simulink model "uz_pmsm_model_6ph_dqxy"  (R2024b)
settings: Solver=FixedStepAuto  StartTime=0.0  StopTime=0.5  RelTol=1e-3
PreLoadFcn:
  | uz_pmsm_model_6ph_dqxy_init_parameter
values from neighbouring files (symbols this model uses):
  friction_coefficient = 0.001    [uz_pmsm_model_6ph_dqxy_init_parameter.m]
  inertia = 0.001    [uz_pmsm_model_6ph_dqxy_init_parameter.m]
  k_i_d = R_1/(2*tau_sum)    (= 10500)    [uz_pmsm_model_6ph_dqxy_init_parameter.m]
  k_i_x = R_1/(2*tau_sum)    (= 10500)    [uz_pmsm_model_6ph_dqxy_init_parameter.m]
  k_i_y = R_1/(2*tau_sum)    (= 10500)    [uz_pmsm_model_6ph_dqxy_init_parameter.m]
  k_p_d = L_d/(2*tau_sum)    (= 150)    [uz_pmsm_model_6ph_dqxy_init_parameter.m]
  k_p_q = L_q/(2*tau_sum)    (= 250)    [uz_pmsm_model_6ph_dqxy_init_parameter.m]
  k_p_x = L_x/(2*tau_sum)    (= 15)    [uz_pmsm_model_6ph_dqxy_init_parameter.m]
  k_p_y = L_y/(2*tau_sum)    (= 25)    [uz_pmsm_model_6ph_dqxy_init_parameter.m]
  L_d = 30e-3    (= 0.03)    [uz_pmsm_model_6ph_dqxy_init_parameter.m]
  L_q = 50e-3    (= 0.05)    [uz_pmsm_model_6ph_dqxy_init_parameter.m]
  L_x = 30e-4    (= 0.003)    [uz_pmsm_model_6ph_dqxy_init_parameter.m]
  L_y = 50e-4    (= 0.005)    [uz_pmsm_model_6ph_dqxy_init_parameter.m]
  polepair = 2    [uz_pmsm_model_6ph_dqxy_init_parameter.m]
  psi_pm = 0.05    [uz_pmsm_model_6ph_dqxy_init_parameter.m]
  R_1 = 2.1    [uz_pmsm_model_6ph_dqxy_init_parameter.m]
  setpoint_step = 10.0    (= 10)    [uz_pmsm_model_6ph_dqxy_init_parameter.m]
  simulate_mechanical = true    [uz_pmsm_model_6ph_dqxy_init_parameter.m]
  simulate_open_loop = true    [uz_pmsm_model_6ph_dqxy_init_parameter.m]
  static_friction_torque = 0.01    [uz_pmsm_model_6ph_dqxy_init_parameter.m]
  ts = 1/2e6    (= 5e-07)    [uz_pmsm_model_6ph_dqxy_init_parameter.m]
libraries: slpidlib x4
settings Model: DataTypeOverride=Off  Creator=ts  LastModifiedBy=hufnagelde
settings SolverCC: AlgebraicLoopSolver=TrustRegion  AutoInsertRateTranBlk=on
settings DataIOCC: LimitDataPoints=on  SaveOutput=off  SaveTime=off
settings OptimizationCC: BlockReduction=off  ConditionallyExecuteInputs=off  DefaultParameterBehavior=Inlined  LifeSpan=inf
settings DebuggingCC: AlgebraicLoopMsg=error  SingleTaskRateTransMsg=error  UnconnectedInputMsg=warning  UnconnectedOutputMsg=warning  UnconnectedLineMsg=warning  AllowSymbolicDim=off  StrictBusMsg=ErrorOnBusTreatedAsVector  SFUnexpectedBacktrackingDiag=warning  SFNoUnconditionalDefaultTransitionDiag=warning  SFExecutionAtInitializationDiag=none  ArithmeticOperatorsInVariantConditions=warning
settings HardwareCC: ProdBitPerPointer=32  ProdBitPerSizeT=32  ProdBitPerPtrDiffT=32  ProdLargestAtomicFloat=None  ProdIntDivRoundTo=Undefined  ProdEndianess=Unspecified  ProdWordSize=32  ProdHWDeviceType=ASIC/FPGA->ASIC/FPGA  ProdEqTarget=off
settings ModelReferenceCC: EnableRefExpFcnMdlSchedulingChecks=on
settings SFSimCC: SimUseLocalCustomCode=off  CustomCodeUndefinedFunction=UseInterfaceOnly
settings RTWCC: RTWUseLocalCustomCode=off  GPUComputeCapability=3.5  DLArmComputeVersion=19.05
settings CodeAppCC: StateflowObjectComments=on
settings GRTTargetCC: TargetLangStandard=C89/C90 (ANSI)
settings ConfigComp: CovScope=ReferencedModels  CovMetricSettings=dw  CovSaveCumulativeToWorkspaceVar=on  CovSaveSingleToWorkspaceVar=on  CovExternalEMLEnable=off  CovSFcnEnable=off

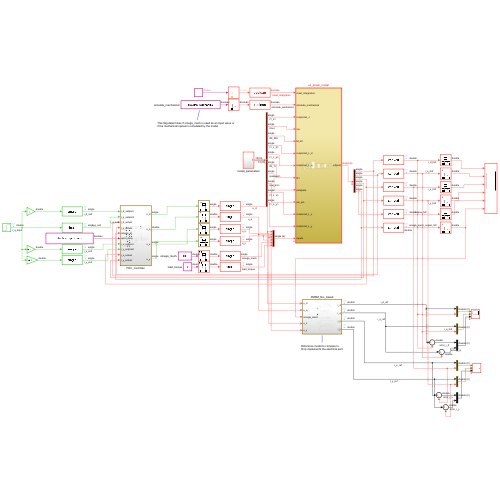
[thumbnail: Simulink's stored preview of the top-level diagram]
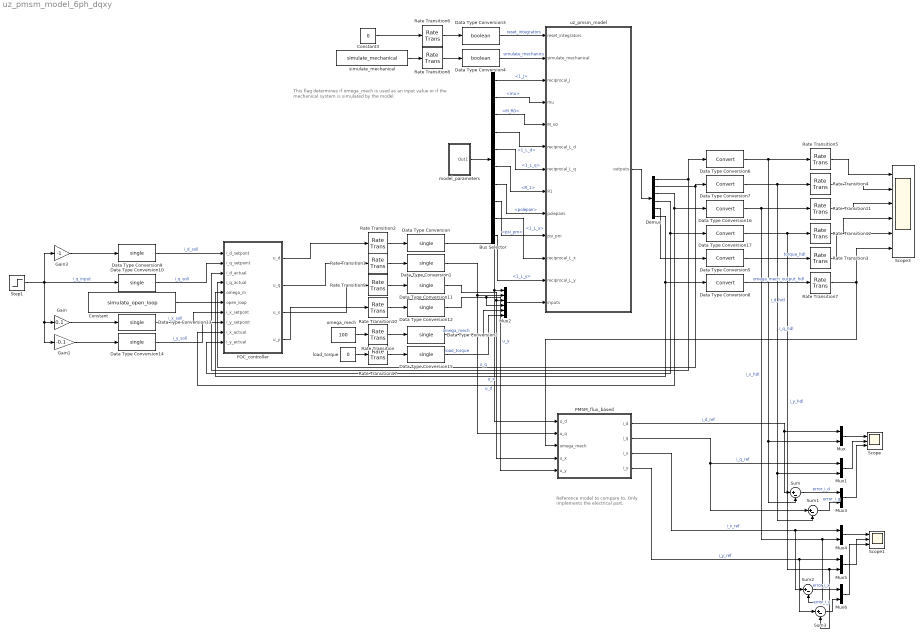
== system uz_pmsm_model_6ph_dqxy ==
  note: Reference model to compare to.
      | Only implements the electrical part.
  note: This flag determines if omega_mech is used as an input value or
      | if the mechanical system is simulated by the model
  Bus Selector : BusSelector  OutputSignals=1_J,mu,M_R0,1_L_d,1_L_q,R_1,polepair,psi_pm,1_L_x,1_L_y
  Constant : Constant  Value=simulate_open_loop
  Constant3 : Constant  Value=0
  Data Type Conversion{,1..2,9..15} (10 alike) : DataTypeConversion  OutDataTypeStr=single  SaturateOnIntegerOverflow=off  RndMeth=Floor
  Data Type Conversion{5..8,16..17} (6 alike) : DataTypeConversion  SaturateOnIntegerOverflow=off  RndMeth=Floor
  Data Type Conversion3 : DataTypeConversion  OutDataTypeStr=boolean  SaturateOnIntegerOverflow=off  RndMeth=Floor
  Data Type Conversion4 : DataTypeConversion  OutDataTypeStr=boolean  SaturateOnIntegerOverflow=off  RndMeth=Floor
  Demux : Demux  Outputs=6
  FOC_controller : Subsystem
  Gain : Gain  Gain=0.1
  Gain1 : Gain  Gain=-0.1
  Gain3 : Gain  Gain=-1
  Mux{,1,3..6} (6 alike) : Mux  Inputs=2
  Mux2 : Mux  Inputs=6
  PMSM_flux_based : Subsystem
  Rate Transition{,1..2,6,8..10,17} (8 alike) : RateTransition  OutPortSampleTime=ts
  Rate Transition{3..5,7,11..12} (6 alike) : RateTransition
  Scope : Scope  NumInputPorts=3
  Scope1 : Scope  NumInputPorts=3
  Scope3 : Scope  NumInputPorts=6
  Step1 : Step  Time=0.2  After=setpoint_step
  Sum{,1..3} (4 alike) : Sum  Inputs=|+-
  load_torque : Constant  Value=0
  model_parameters : Subsystem
  omega_mech : Constant  Value=100
  simulate_mechanical : Constant  Value=simulate_mechanical
  uz_pmsm_model : Subsystem  TreatAsAtomicUnit=on
  wires:
  Rate Transition/1 -> Data Type Conversion2/1
  Data Type Conversion6/1 -> Mux/2, Sum/2, Rate Transition5/1  "i_d_hdl"
  Data Type Conversion7/1 -> Mux1/2, Sum1/2, Rate Transition4/1  "i_q_hdl"
  Data Type Conversion5/1 -> Rate Transition3/1  "torque_hdl"
  Rate Transition4/1 -> Scope3/2
  Rate Transition5/1 -> Scope3/1
  Rate Transition3/1 -> Scope3/5
  Rate Transition6/1 -> Data Type Conversion3/1
  Constant3/1 -> Rate Transition6/1
  Rate Transition8/1 -> Data Type Conversion4/1
  simulate_mechanical/1 -> Rate Transition8/1
  Data Type Conversion3/1 -> uz_pmsm_model/1(reset_integrators)  "reset_integrators"
  Data Type Conversion4/1 -> uz_pmsm_model/2(simulate_mechanical)  "simulate_mechanics"
  load_torque/1 -> Rate Transition17/1
  Rate Transition17/1 -> Data Type Conversion15/1
  Mux/1 -> Scope/1
  Mux1/1 -> Scope/2
  PMSM_flux_based/2(i_q) -> Mux1/1, Sum1/1  "i_q_ref"
  PMSM_flux_based/1(i_d) -> Mux/1, Sum/1  "i_d_ref"
  Data Type Conversion8/1 -> Rate Transition7/1  "omega_mech_output_hdl"
  Rate Transition7/1 -> PMSM_flux_based/3(omega_mech), Scope3/6
  Bus Selector/1 -> uz_pmsm_model/3(reciprocal_J)  "<1_J>"
  Bus Selector/2 -> uz_pmsm_model/4(mu)  "<mu>"
  Bus Selector/3 -> uz_pmsm_model/5(M_n0)  "<M_R0>"
  Bus Selector/4 -> uz_pmsm_model/6(reciprocal_L_d)  "<1_L_d>"
  Bus Selector/5 -> uz_pmsm_model/7(reciprocal_L_q)  "<1_L_q>"
  Bus Selector/6 -> uz_pmsm_model/8(R1)  "<R_1>"
  Bus Selector/7 -> uz_pmsm_model/9(polepairs)  "<polepair>"
  Bus Selector/8 -> uz_pmsm_model/10(psi_pm)  "<psi_pm>"
  model_parameters/1(Out1) -> Bus Selector/1
  Sum/1 -> Mux3/1  "error_i_d"
  Sum1/1 -> Mux3/2  "error_i_q"
  Mux3/1 -> Scope/3
  Step1/1 -> Gain1/1, Gain/1, Gain3/1, Data Type Conversion10/1  "i_q_input"
  Demux/5 -> Data Type Conversion5/1
  Gain3/1 -> Data Type Conversion9/1
  Demux/1 -> FOC_controller/3(i_d_actual), Data Type Conversion6/1
  Demux/6 -> FOC_controller/5(omega_m), Data Type Conversion8/1
  Demux/2 -> FOC_controller/4(i_q_actual), Data Type Conversion7/1
  Data Type Conversion/1 -> PMSM_flux_based/1(u_d), Mux2/1  "u_d"
  Data Type Conversion1/1 -> PMSM_flux_based/2(u_q), Mux2/2  "u_q"
  Data Type Conversion15/1 -> Mux2/6  "load_torque"
  Data Type Conversion2/1 -> Mux2/5  "omega_mech"
  Mux2/1 -> uz_pmsm_model/13(inputs)
  uz_pmsm_model/1(outputs) -> Demux/1
  Data Type Conversion9/1 -> FOC_controller/1(i_d_setpont)  "i_d_soll"
  Data Type Conversion10/1 -> FOC_controller/2(i_q_setpoint)  "i_q_soll"
  omega_mech/1 -> Rate Transition/1
  Constant/1 -> FOC_controller/6(open_loop)
  Rate Transition9/1 -> Data Type Conversion11/1
  Rate Transition10/1 -> Data Type Conversion12/1
  Rate Transition1/1 -> Data Type Conversion1/1
  Rate Transition2/1 -> Data Type Conversion/1
  FOC_controller/1(u_d) -> Rate Transition2/1
  FOC_controller/2(u_q) -> Rate Transition1/1
  FOC_controller/3(u_x) -> Rate Transition9/1
  FOC_controller/4(u_y) -> Rate Transition10/1
  Data Type Conversion11/1 -> PMSM_flux_based/4(u_x), Mux2/3  "u_x"
  Data Type Conversion12/1 -> PMSM_flux_based/5(u_y), Mux2/4  "u_y"
  Gain1/1 -> Data Type Conversion14/1
  Gain/1 -> Data Type Conversion13/1
  Data Type Conversion13/1 -> FOC_controller/7(i_x_setpont)  "i_x_soll"
  Data Type Conversion14/1 -> FOC_controller/8(i_y_setpoint)  "i_y_soll"
  Data Type Conversion16/1 -> Sum2/2, Mux4/2, Rate Transition11/1  "i_x_hdl"
  Rate Transition11/1 -> Scope3/3
  Demux/3 -> FOC_controller/9(i_x_actual), Data Type Conversion16/1
  Data Type Conversion17/1 -> Sum3/2, Mux5/2, Rate Transition12/1  "i_y_hdl"
  Rate Transition12/1 -> Scope3/4
  Demux/4 -> FOC_controller/10(i_y_actual), Data Type Conversion17/1
  Mux4/1 -> Scope1/1
  PMSM_flux_based/3(i_x) -> Sum2/1, Mux4/1  "i_x_ref"
  PMSM_flux_based/4(i_y) -> Mux5/1, Sum3/1  "i_y_ref"
  Mux5/1 -> Scope1/2
  Sum2/1 -> Mux6/1  "error_i_x"
  Sum3/1 -> Mux6/2  "error_i_y"
  Mux6/1 -> Scope1/3
  Bus Selector/9 -> uz_pmsm_model/11(reciprocal_L_x)  "<1_L_x>"
  Bus Selector/10 -> uz_pmsm_model/12(reciprocal_L_y)  "<1_L_y>"

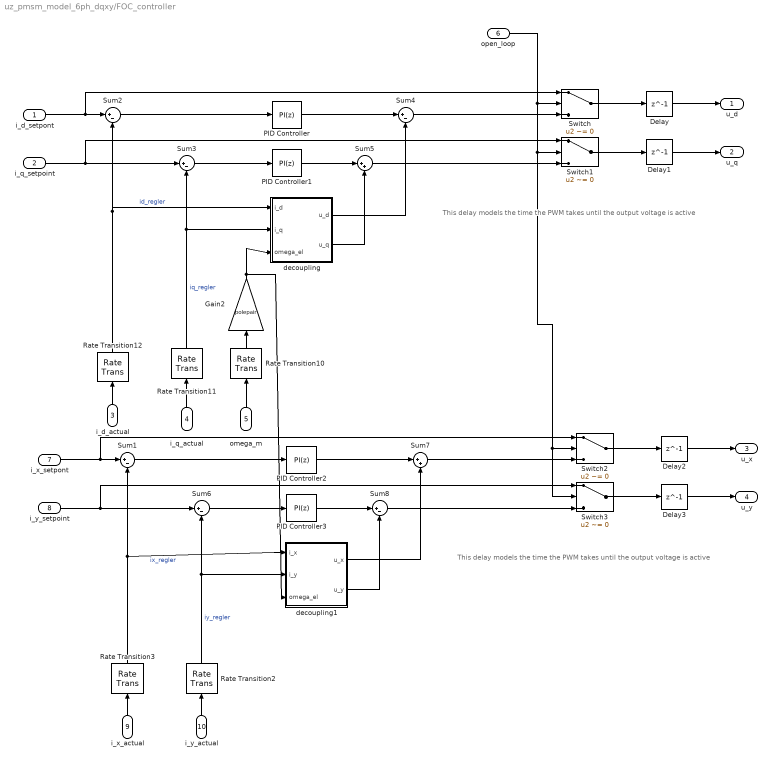
== system uz_pmsm_model_6ph_dqxy/FOC_controller ==
  note: This delay models the time the PWM takes until the output voltage is active
  note: This delay models the time the PWM takes until the output voltage is active
  i_d_setpont : Inport
  i_q_setpoint : Inport  Port=2
  i_d_actual : Inport  Port=3
  i_q_actual : Inport  Port=4
  omega_m : Inport  Port=5
  open_loop : Inport  Port=6
  i_x_setpont : Inport  Port=7
  i_y_setpoint : Inport  Port=8
  i_x_actual : Inport  Port=9
  i_y_actual : Inport  Port=10
  Delay{,1..3} (4 alike) : Delay  DelayLength=1
  Gain2 : Gain  Gain=polepair
  PID Controller : slpidlib/PID Controller  Controller=PI  Form=Parallel  TimeDomain=Discrete-time  UseExternalTs=off  SampleTime=-1  IntegratorMethod=Forward Euler  FilterMethod=Forward Euler  ControllerParametersSource=internal  P=k_p_d  I=k_i_d  UseKiTs=off  D=0  UseExternalDerivativeSource=off  N=100  UseFilter=on  TunerSelectOption=Transfer Function Based (PID Tuner App)  InitialConditionSource=internal  InitialConditionForIntegrator=0  InitialConditionForFilter=0  DifferentiatorICPrevScaledInput=0  ExternalReset=none  TrackingMode=off  Kt=1  LimitOutput=off  SatLimitsSource=internal  UpperSaturationLimit=inf  LowerSaturationLimit=-inf  LinearizeAsGain=on  AntiWindupMode=none  Kb=1  LimitIntegrator=off  UpperIntegratorSaturationLimit=inf  LowerIntegratorSaturationLimit=-inf  POutMin=[]  POutMax=[]  IOutMin=[]  IOutMax=[]  DOutMin=[]  DOutMax=[]  NOutMin=[]  NOutMax=[]  SumOutMin=[]  SumOutMax=[]  SaturationOutMin=[]  SaturationOutMax=[]  PParamMin=[]  PParamMax=[]  IParamMin=[]  IParamMax=[]  DParamMin=[]  DParamMax=[]  NParamMin=[]  NParamMax=[]  KbParamMin=[]  KbParamMax=[]  KtParamMin=[]  KtParamMax=[]  KbOutMin=[]  KbOutMax=[]  KtOutMin=[]  KtOutMax=[]  IntegratorOutMin=[]  IntegratorOutMax=[]  FilterOutMin=[]  FilterOutMax=[]  SumI1OutMin=[]  SumI1OutMax=[]  SumI2OutMin=[]  SumI2OutMax=[]  SumI3OutMin=[]  SumI3OutMax=[]  SumI4OutMin=[]  SumI4OutMax=[]  SumDOutMin=[]  SumDOutMax=[]  DifferentiatorOutMin=[]  DifferentiatorOutMax=[]  FilterDiffOutCoefMin=[]  FilterDiffOutCoefMax=[]  ReciprocalOutMin=[]  ReciprocalOutMax=[]  SumDenOutMin=[]  SumDenOutMax=[]  SumNumOutMin=[]  SumNumOutMax=[]  DivideOutMin=[]  DivideOutMax=[]  UdiffTsProdOutMin=[]  UdiffTsProdOutMax=[]  NTsProdOutMin=[]  NTsProdOutMax=[]  UintegralTsProdOutMin=[]  UintegralTsProdOutMax=[]  UngainTsProdOutMin=[]  UngainTsProdOutMax=[]  ClampingZeroOutDataTypeStr=Inherit: Inherit via back propagation  ClampingZeroOutMin=[]  ClampingZeroOutMax=[]  FilterDenConstantOutDataTypeStr=Inherit: Inherit via back propagation  FilterDenConstantOutMin=[]  FilterDenConstantOutMax=[]  PCopyOutDataTypeStr=Inherit: Inherit via back propagation  PCopyOutMin=[]  PCopyOutMax=[]  NCopyOutDataTypeStr=Inherit: Inherit via back propagation  NCopyOutMin=[]  NCopyOutMax=[]  IntegratorContinuousStateAttributes=''  IntegratorStateMustResolveToSignalObject=off  IntegratorRTWStateStorageClass=Auto  FilterContinuousStateAttributes=''  FilterStateMustResolveToSignalObject=off  FilterRTWStateStorageClass=Auto  ParallelPVariant=InternalParameters  IdealPVariant=Disabled  IVariant=InternalParameters  DVariant=Disabled  IntegratorVariant=Discrete  SatVariant=Disabled  AWVariant=Passthrough  PCopyVariant=Disabled  TRVariant=Disabled  FdbkBlocksVariant=Forward  IdealPFdbkVariant=Disabled  SatFdbkVariant=Disabled  DerivativeFilterVariant=Disabled  NVariant=Disabled  NCopyVariant=Disabled_SignalSpec  FilterICVariant=Disabled  IntegratorICVariant=InternalICs  ExternalResetVariant=Disabled  TRSumVariant=Passthrough  SumFdbkVariant=Disabled  SumVariant=Sum_PI  TsampFilterVariant=InternalTs  TsampNgainVariant=Passthrough  TsampIntegralVariant=Disabled_SignalSpec  ExternalSaturationOutDataTypeStr=Inherit: Same as second input  DerivativeSourceVariant=Disabled  PreIntVariant=InternalPreInt
  PID Controller1 : slpidlib/PID Controller  Controller=PI  Form=Parallel  TimeDomain=Discrete-time  UseExternalTs=off  SampleTime=-1  IntegratorMethod=Forward Euler  FilterMethod=Forward Euler  ControllerParametersSource=internal  P=k_p_q  I=k_i_d  UseKiTs=off  D=0  UseExternalDerivativeSource=off  N=100  UseFilter=on  TunerSelectOption=Transfer Function Based (PID Tuner App)  InitialConditionSource=internal  InitialConditionForIntegrator=0  InitialConditionForFilter=0  DifferentiatorICPrevScaledInput=0  ExternalReset=none  TrackingMode=off  Kt=1  LimitOutput=off  SatLimitsSource=internal  UpperSaturationLimit=inf  LowerSaturationLimit=-inf  LinearizeAsGain=on  AntiWindupMode=none  Kb=1  LimitIntegrator=off  UpperIntegratorSaturationLimit=inf  LowerIntegratorSaturationLimit=-inf  POutMin=[]  POutMax=[]  IOutMin=[]  IOutMax=[]  DOutMin=[]  DOutMax=[]  NOutMin=[]  NOutMax=[]  SumOutMin=[]  SumOutMax=[]  SaturationOutMin=[]  SaturationOutMax=[]  PParamMin=[]  PParamMax=[]  IParamMin=[]  IParamMax=[]  DParamMin=[]  DParamMax=[]  NParamMin=[]  NParamMax=[]  KbParamMin=[]  KbParamMax=[]  KtParamMin=[]  KtParamMax=[]  KbOutMin=[]  KbOutMax=[]  KtOutMin=[]  KtOutMax=[]  IntegratorOutMin=[]  IntegratorOutMax=[]  FilterOutMin=[]  FilterOutMax=[]  SumI1OutMin=[]  SumI1OutMax=[]  SumI2OutMin=[]  SumI2OutMax=[]  SumI3OutMin=[]  SumI3OutMax=[]  SumI4OutMin=[]  SumI4OutMax=[]  SumDOutMin=[]  SumDOutMax=[]  DifferentiatorOutMin=[]  DifferentiatorOutMax=[]  FilterDiffOutCoefMin=[]  FilterDiffOutCoefMax=[]  ReciprocalOutMin=[]  ReciprocalOutMax=[]  SumDenOutMin=[]  SumDenOutMax=[]  SumNumOutMin=[]  SumNumOutMax=[]  DivideOutMin=[]  DivideOutMax=[]  UdiffTsProdOutMin=[]  UdiffTsProdOutMax=[]  NTsProdOutMin=[]  NTsProdOutMax=[]  UintegralTsProdOutMin=[]  UintegralTsProdOutMax=[]  UngainTsProdOutMin=[]  UngainTsProdOutMax=[]  ClampingZeroOutDataTypeStr=Inherit: Inherit via back propagation  ClampingZeroOutMin=[]  ClampingZeroOutMax=[]  FilterDenConstantOutDataTypeStr=Inherit: Inherit via back propagation  FilterDenConstantOutMin=[]  FilterDenConstantOutMax=[]  PCopyOutDataTypeStr=Inherit: Inherit via back propagation  PCopyOutMin=[]  PCopyOutMax=[]  NCopyOutDataTypeStr=Inherit: Inherit via back propagation  NCopyOutMin=[]  NCopyOutMax=[]  IntegratorContinuousStateAttributes=''  IntegratorStateMustResolveToSignalObject=off  IntegratorRTWStateStorageClass=Auto  FilterContinuousStateAttributes=''  FilterStateMustResolveToSignalObject=off  FilterRTWStateStorageClass=Auto  ParallelPVariant=InternalParameters  IdealPVariant=Disabled  IVariant=InternalParameters  DVariant=Disabled  IntegratorVariant=Discrete  SatVariant=Disabled  AWVariant=Passthrough  PCopyVariant=Disabled  TRVariant=Disabled  FdbkBlocksVariant=Forward  IdealPFdbkVariant=Disabled  SatFdbkVariant=Disabled  DerivativeFilterVariant=Disabled  NVariant=Disabled  NCopyVariant=Disabled_SignalSpec  FilterICVariant=Disabled  IntegratorICVariant=InternalICs  ExternalResetVariant=Disabled  TRSumVariant=Passthrough  SumFdbkVariant=Disabled  SumVariant=Sum_PI  TsampFilterVariant=InternalTs  TsampNgainVariant=Passthrough  TsampIntegralVariant=Disabled_SignalSpec  ExternalSaturationOutDataTypeStr=Inherit: Same as second input  DerivativeSourceVariant=Disabled  PreIntVariant=InternalPreInt
  PID Controller2 : slpidlib/PID Controller  Controller=PI  Form=Parallel  TimeDomain=Discrete-time  UseExternalTs=off  SampleTime=-1  IntegratorMethod=Forward Euler  FilterMethod=Forward Euler  ControllerParametersSource=internal  P=k_p_x  I=k_i_x  UseKiTs=off  D=0  UseExternalDerivativeSource=off  N=100  UseFilter=on  TunerSelectOption=Transfer Function Based (PID Tuner App)  InitialConditionSource=internal  InitialConditionForIntegrator=0  InitialConditionForFilter=0  DifferentiatorICPrevScaledInput=0  ExternalReset=none  TrackingMode=off  Kt=1  LimitOutput=off  SatLimitsSource=internal  UpperSaturationLimit=inf  LowerSaturationLimit=-inf  LinearizeAsGain=on  AntiWindupMode=none  Kb=1  LimitIntegrator=off  UpperIntegratorSaturationLimit=inf  LowerIntegratorSaturationLimit=-inf  POutMin=[]  POutMax=[]  IOutMin=[]  IOutMax=[]  DOutMin=[]  DOutMax=[]  NOutMin=[]  NOutMax=[]  SumOutMin=[]  SumOutMax=[]  SaturationOutMin=[]  SaturationOutMax=[]  PParamMin=[]  PParamMax=[]  IParamMin=[]  IParamMax=[]  DParamMin=[]  DParamMax=[]  NParamMin=[]  NParamMax=[]  KbParamMin=[]  KbParamMax=[]  KtParamMin=[]  KtParamMax=[]  KbOutMin=[]  KbOutMax=[]  KtOutMin=[]  KtOutMax=[]  IntegratorOutMin=[]  IntegratorOutMax=[]  FilterOutMin=[]  FilterOutMax=[]  SumI1OutMin=[]  SumI1OutMax=[]  SumI2OutMin=[]  SumI2OutMax=[]  SumI3OutMin=[]  SumI3OutMax=[]  SumI4OutMin=[]  SumI4OutMax=[]  SumDOutMin=[]  SumDOutMax=[]  DifferentiatorOutMin=[]  DifferentiatorOutMax=[]  FilterDiffOutCoefMin=[]  FilterDiffOutCoefMax=[]  ReciprocalOutMin=[]  ReciprocalOutMax=[]  SumDenOutMin=[]  SumDenOutMax=[]  SumNumOutMin=[]  SumNumOutMax=[]  DivideOutMin=[]  DivideOutMax=[]  UdiffTsProdOutMin=[]  UdiffTsProdOutMax=[]  NTsProdOutMin=[]  NTsProdOutMax=[]  UintegralTsProdOutMin=[]  UintegralTsProdOutMax=[]  UngainTsProdOutMin=[]  UngainTsProdOutMax=[]  ClampingZeroOutDataTypeStr=Inherit: Inherit via back propagation  ClampingZeroOutMin=[]  ClampingZeroOutMax=[]  FilterDenConstantOutDataTypeStr=Inherit: Inherit via back propagation  FilterDenConstantOutMin=[]  FilterDenConstantOutMax=[]  PCopyOutDataTypeStr=Inherit: Inherit via back propagation  PCopyOutMin=[]  PCopyOutMax=[]  NCopyOutDataTypeStr=Inherit: Inherit via back propagation  NCopyOutMin=[]  NCopyOutMax=[]  IntegratorContinuousStateAttributes=''  IntegratorStateMustResolveToSignalObject=off  IntegratorRTWStateStorageClass=Auto  FilterContinuousStateAttributes=''  FilterStateMustResolveToSignalObject=off  FilterRTWStateStorageClass=Auto  ParallelPVariant=InternalParameters  IdealPVariant=Disabled  IVariant=InternalParameters  DVariant=Disabled  IntegratorVariant=Discrete  SatVariant=Disabled  AWVariant=Passthrough  PCopyVariant=Disabled  TRVariant=Disabled  FdbkBlocksVariant=Forward  IdealPFdbkVariant=Disabled  SatFdbkVariant=Disabled  DerivativeFilterVariant=Disabled  NVariant=Disabled  NCopyVariant=Disabled_SignalSpec  FilterICVariant=Disabled  IntegratorICVariant=InternalICs  ExternalResetVariant=Disabled  TRSumVariant=Passthrough  SumFdbkVariant=Disabled  SumVariant=Sum_PI  TsampFilterVariant=InternalTs  TsampNgainVariant=Passthrough  TsampIntegralVariant=Disabled_SignalSpec  ExternalSaturationOutDataTypeStr=Inherit: Same as second input  DerivativeSourceVariant=Disabled  PreIntVariant=InternalPreInt
  PID Controller3 : slpidlib/PID Controller  Controller=PI  Form=Parallel  TimeDomain=Discrete-time  UseExternalTs=off  SampleTime=-1  IntegratorMethod=Forward Euler  FilterMethod=Forward Euler  ControllerParametersSource=internal  P=k_p_y  I=k_i_y  UseKiTs=off  D=0  UseExternalDerivativeSource=off  N=100  UseFilter=on  TunerSelectOption=Transfer Function Based (PID Tuner App)  InitialConditionSource=internal  InitialConditionForIntegrator=0  InitialConditionForFilter=0  DifferentiatorICPrevScaledInput=0  ExternalReset=none  TrackingMode=off  Kt=1  LimitOutput=off  SatLimitsSource=internal  UpperSaturationLimit=inf  LowerSaturationLimit=-inf  LinearizeAsGain=on  AntiWindupMode=none  Kb=1  LimitIntegrator=off  UpperIntegratorSaturationLimit=inf  LowerIntegratorSaturationLimit=-inf  POutMin=[]  POutMax=[]  IOutMin=[]  IOutMax=[]  DOutMin=[]  DOutMax=[]  NOutMin=[]  NOutMax=[]  SumOutMin=[]  SumOutMax=[]  SaturationOutMin=[]  SaturationOutMax=[]  PParamMin=[]  PParamMax=[]  IParamMin=[]  IParamMax=[]  DParamMin=[]  DParamMax=[]  NParamMin=[]  NParamMax=[]  KbParamMin=[]  KbParamMax=[]  KtParamMin=[]  KtParamMax=[]  KbOutMin=[]  KbOutMax=[]  KtOutMin=[]  KtOutMax=[]  IntegratorOutMin=[]  IntegratorOutMax=[]  FilterOutMin=[]  FilterOutMax=[]  SumI1OutMin=[]  SumI1OutMax=[]  SumI2OutMin=[]  SumI2OutMax=[]  SumI3OutMin=[]  SumI3OutMax=[]  SumI4OutMin=[]  SumI4OutMax=[]  SumDOutMin=[]  SumDOutMax=[]  DifferentiatorOutMin=[]  DifferentiatorOutMax=[]  FilterDiffOutCoefMin=[]  FilterDiffOutCoefMax=[]  ReciprocalOutMin=[]  ReciprocalOutMax=[]  SumDenOutMin=[]  SumDenOutMax=[]  SumNumOutMin=[]  SumNumOutMax=[]  DivideOutMin=[]  DivideOutMax=[]  UdiffTsProdOutMin=[]  UdiffTsProdOutMax=[]  NTsProdOutMin=[]  NTsProdOutMax=[]  UintegralTsProdOutMin=[]  UintegralTsProdOutMax=[]  UngainTsProdOutMin=[]  UngainTsProdOutMax=[]  ClampingZeroOutDataTypeStr=Inherit: Inherit via back propagation  ClampingZeroOutMin=[]  ClampingZeroOutMax=[]  FilterDenConstantOutDataTypeStr=Inherit: Inherit via back propagation  FilterDenConstantOutMin=[]  FilterDenConstantOutMax=[]  PCopyOutDataTypeStr=Inherit: Inherit via back propagation  PCopyOutMin=[]  PCopyOutMax=[]  NCopyOutDataTypeStr=Inherit: Inherit via back propagation  NCopyOutMin=[]  NCopyOutMax=[]  IntegratorContinuousStateAttributes=''  IntegratorStateMustResolveToSignalObject=off  IntegratorRTWStateStorageClass=Auto  FilterContinuousStateAttributes=''  FilterStateMustResolveToSignalObject=off  FilterRTWStateStorageClass=Auto  ParallelPVariant=InternalParameters  IdealPVariant=Disabled  IVariant=InternalParameters  DVariant=Disabled  IntegratorVariant=Discrete  SatVariant=Disabled  AWVariant=Passthrough  PCopyVariant=Disabled  TRVariant=Disabled  FdbkBlocksVariant=Forward  IdealPFdbkVariant=Disabled  SatFdbkVariant=Disabled  DerivativeFilterVariant=Disabled  NVariant=Disabled  NCopyVariant=Disabled_SignalSpec  FilterICVariant=Disabled  IntegratorICVariant=InternalICs  ExternalResetVariant=Disabled  TRSumVariant=Passthrough  SumFdbkVariant=Disabled  SumVariant=Sum_PI  TsampFilterVariant=InternalTs  TsampNgainVariant=Passthrough  TsampIntegralVariant=Disabled_SignalSpec  ExternalSaturationOutDataTypeStr=Inherit: Same as second input  DerivativeSourceVariant=Disabled  PreIntVariant=InternalPreInt
  Rate Transition{2..3,10..12} (5 alike) : RateTransition  OutPortSampleTime=ts_regler
  Sum{1..4,6,8} (6 alike) : Sum  Inputs=|+-
  Sum5 : Sum  Inputs=|++
  Sum7 : Sum  Inputs=|++
  Switch{,1..3} (4 alike) : Switch  Criteria=u2 ~= 0  SaturateOnIntegerOverflow=off  InputSameDT=off
  decoupling : Subsystem
  decoupling1 : Subsystem
  u_d : Outport
  u_q : Outport  Port=2
  u_x : Outport  Port=3
  u_y : Outport  Port=4
  wires:
  PID Controller/1 -> Sum4/1
  PID Controller1/1 -> Sum5/1
  Sum4/1 -> Switch/3
  i_d_actual/1 -> Rate Transition12/1
  i_d_setpont/1 -> Switch/1, Sum2/1
  Sum2/1 -> PID Controller/1
  Sum5/1 -> Switch1/3
  Sum3/1 -> PID Controller1/1
  i_q_actual/1 -> Rate Transition11/1
  Rate Transition12/1 -> decoupling/1(i_d), Sum2/2  "id_regler"
  Rate Transition11/1 -> decoupling/2(i_q), Sum3/2  "iq_regler"
  i_q_setpoint/1 -> Switch1/1, Sum3/1
  Rate Transition10/1 -> Gain2/1
  decoupling/1(u_d) -> Sum4/2
  decoupling/2(u_q) -> Sum5/2
  Switch/1 -> Delay/1
  Switch1/1 -> Delay1/1
  Delay/1 -> u_d/1
  Delay1/1 -> u_q/1
  Switch2/1 -> Delay2/1
  PID Controller3/1 -> Sum8/1
  Sum1/1 -> PID Controller2/1
  omega_m/1 -> Rate Transition10/1
  Delay2/1 -> u_x/1
  PID Controller2/1 -> Sum7/1
  Delay3/1 -> u_y/1
  Sum8/1 -> Switch3/3
  Sum6/1 -> PID Controller3/1
  Sum7/1 -> Switch2/3
  i_x_actual/1 -> Rate Transition3/1
  open_loop/1 -> Switch3/2, Switch2/2, Switch1/2, Switch/2
  i_y_setpoint/1 -> Switch3/1, Sum6/1
  i_y_actual/1 -> Rate Transition2/1
  Rate Transition2/1 -> decoupling1/2(i_y), Sum6/2  "iy_regler"
  decoupling1/2(u_y) -> Sum8/2
  i_x_setpont/1 -> Switch2/1, Sum1/1
  Switch3/1 -> Delay3/1
  Rate Transition3/1 -> decoupling1/1(i_x), Sum1/2  "ix_regler"
  decoupling1/1(u_x) -> Sum7/2
  Gain2/1 -> decoupling1/3(omega_el), decoupling/3(omega_el)

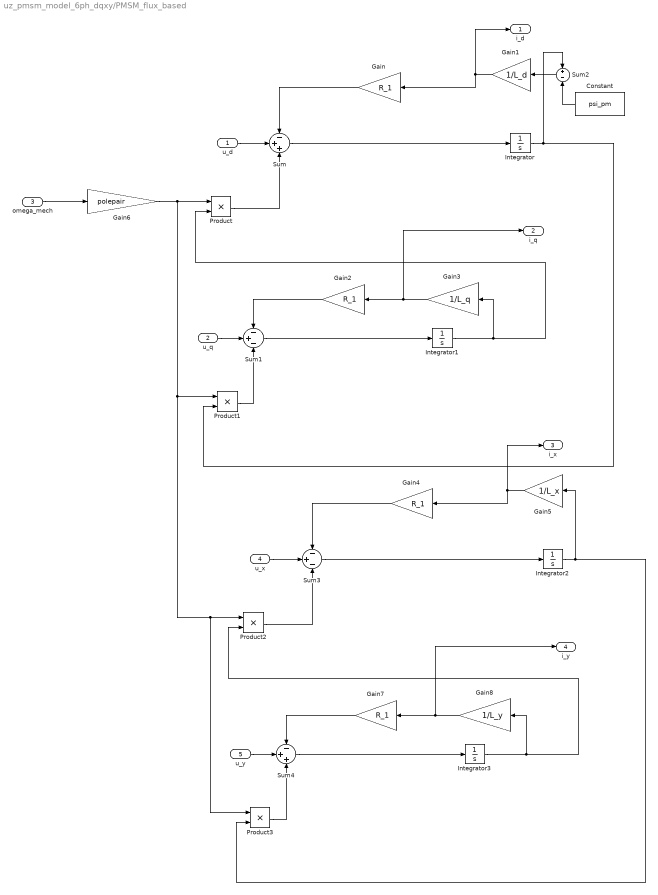
== system uz_pmsm_model_6ph_dqxy/PMSM_flux_based ==
  u_d : Inport
  u_q : Inport  Port=2
  omega_mech : Inport  Port=3
  u_x : Inport  Port=4
  u_y : Inport  Port=5
  Constant : Constant  Value=psi_pm
  Gain{,2,4,7} (4 alike) : Gain  Gain=R_1
  Gain1 : Gain  Gain=1/L_d
  Gain3 : Gain  Gain=1/L_q
  Gain5 : Gain  Gain=1/L_x
  Gain6 : Gain  Gain=polepair
  Gain8 : Gain  Gain=1/L_y
  Integrator{,1..3} (4 alike) : Integrator
  Product{,1..3} (4 alike) : Product
  Sum : Sum  Inputs=-++
  Sum1 : Sum  Inputs=-+-
  Sum2 : Sum  Inputs=+-
  Sum3 : Sum  Inputs=-+-
  Sum4 : Sum  Inputs=-++
  i_d : Outport
  i_q : Outport  Port=2
  i_x : Outport  Port=3
  i_y : Outport  Port=4
  wires:
  u_d/1 -> Sum/2
  u_q/1 -> Sum1/2
  Sum/1 -> Integrator/1
  Gain/1 -> Sum/1
  Integrator/1 -> Product1/2, Sum2/1
  Constant/1 -> Sum2/2
  Sum2/1 -> Gain1/1
  Gain1/1 -> Gain/1, i_d/1
  Product/1 -> Sum/3
  Integrator1/1 -> Gain3/1, Product/2
  Product1/1 -> Sum1/3
  Sum1/1 -> Integrator1/1
  Gain2/1 -> Sum1/1
  Gain3/1 -> i_q/1, Gain2/1
  omega_mech/1 -> Gain6/1
  Gain5/1 -> Gain4/1, i_x/1
  Sum4/1 -> Integrator3/1
  Product3/1 -> Sum4/3
  Gain8/1 -> i_y/1, Gain7/1
  Gain6/1 -> Product3/1, Product2/1, Product1/1, Product/1
  Sum3/1 -> Integrator2/1
  Product2/1 -> Sum3/3
  Gain4/1 -> Sum3/1
  Integrator3/1 -> Gain8/1, Product2/2
  u_x/1 -> Sum3/2
  u_y/1 -> Sum4/2
  Gain7/1 -> Sum4/1
  Integrator2/1 -> Gain5/1, Product3/2

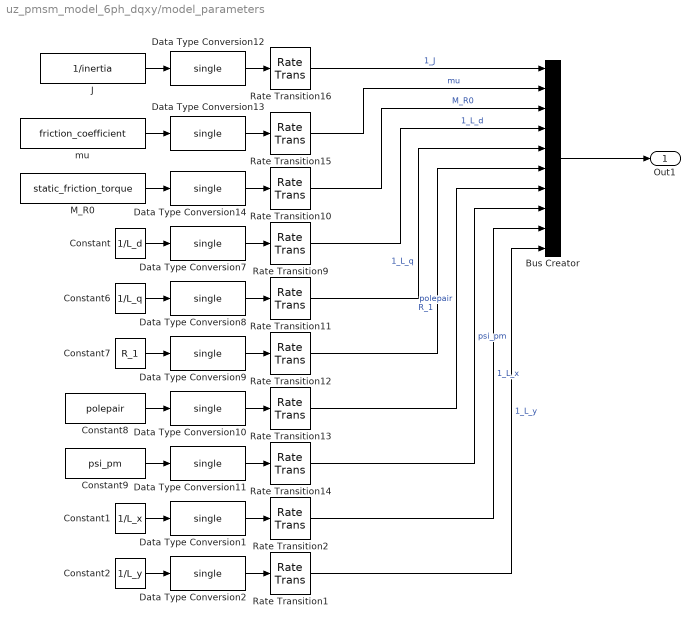
== system uz_pmsm_model_6ph_dqxy/model_parameters ==
  Bus Creator : BusCreator  Inputs=10
  Constant : Constant  Value=1/L_d
  Constant1 : Constant  Value=1/L_x
  Constant2 : Constant  Value=1/L_y
  Constant6 : Constant  Value=1/L_q
  Constant7 : Constant  Value=R_1
  Constant8 : Constant  Value=polepair
  Constant9 : Constant  Value=psi_pm
  Data Type Conversion{1..2,7..14} (10 alike) : DataTypeConversion  OutDataTypeStr=single  SaturateOnIntegerOverflow=off  RndMeth=Floor
  J : Constant  Value=1/inertia
  M_R0 : Constant  Value=static_friction_torque
  Rate Transition{1..2,9..16} (10 alike) : RateTransition  OutPortSampleTime=ts
  mu : Constant  Value=friction_coefficient
  Out1 : Outport
  wires:
  Data Type Conversion12/1 -> Rate Transition16/1
  Data Type Conversion7/1 -> Rate Transition9/1
  Rate Transition10/1 -> Bus Creator/3  "M_R0"
  Rate Transition14/1 -> Bus Creator/8  "psi_pm"
  Data Type Conversion14/1 -> Rate Transition10/1
  Rate Transition12/1 -> Bus Creator/6  "R_1"
  Rate Transition16/1 -> Bus Creator/1  "1_J"
  Rate Transition13/1 -> Bus Creator/7  "polepair"
  Bus Creator/1 -> Out1/1
  Data Type Conversion11/1 -> Rate Transition14/1
  Constant8/1 -> Data Type Conversion10/1
  Data Type Conversion9/1 -> Rate Transition12/1
  Rate Transition15/1 -> Bus Creator/2  "mu"
  Constant6/1 -> Data Type Conversion8/1
  Rate Transition9/1 -> Bus Creator/4  "1_L_d"
  J/1 -> Data Type Conversion12/1
  Data Type Conversion8/1 -> Rate Transition11/1
  Data Type Conversion10/1 -> Rate Transition13/1
  mu/1 -> Data Type Conversion13/1
  M_R0/1 -> Data Type Conversion14/1
  Rate Transition11/1 -> Bus Creator/5  "1_L_q"
  Data Type Conversion13/1 -> Rate Transition15/1
  Constant7/1 -> Data Type Conversion9/1
  Constant9/1 -> Data Type Conversion11/1
  Constant/1 -> Data Type Conversion7/1
  Constant1/1 -> Data Type Conversion1/1
  Constant2/1 -> Data Type Conversion2/1
  Data Type Conversion1/1 -> Rate Transition2/1
  Data Type Conversion2/1 -> Rate Transition1/1
  Rate Transition2/1 -> Bus Creator/9  "1_L_x"
  Rate Transition1/1 -> Bus Creator/10  "1_L_y"

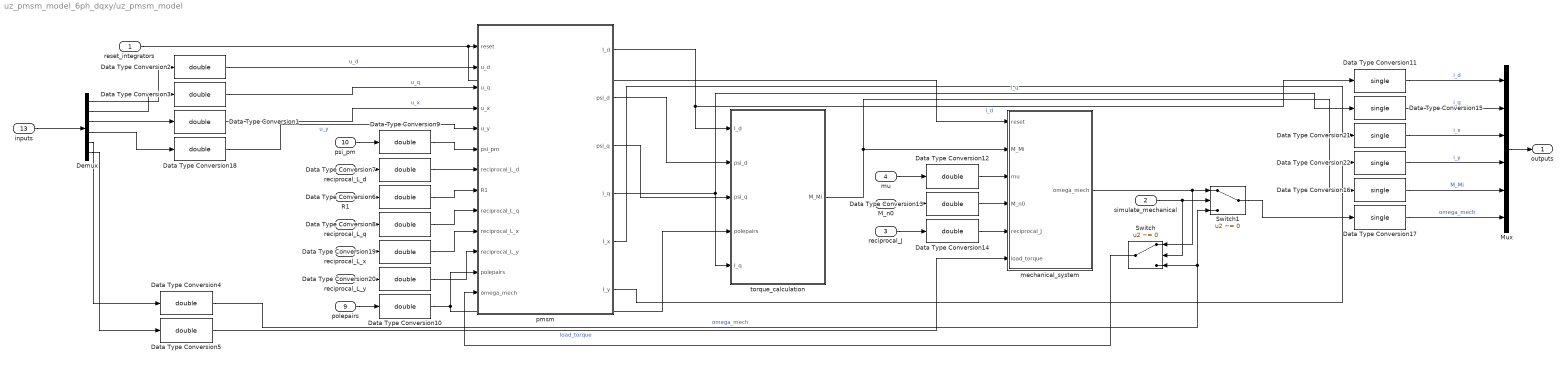
== system uz_pmsm_model_6ph_dqxy/uz_pmsm_model ==
  reset_integrators : Inport
  simulate_mechanical : Inport  Port=2
  reciprocal_J : Inport  Port=3
  mu : Inport  Port=4
  M_n0 : Inport  Port=5
  reciprocal_L_d : Inport  Port=6
  reciprocal_L_q : Inport  Port=7
  R1 : Inport  Port=8
  polepairs : Inport  Port=9
  psi_pm : Inport  Port=10
  reciprocal_L_x : Inport  Port=11
  reciprocal_L_y : Inport  Port=12
  inputs : Inport  Port=13
  Data Type Conversion{1..10,12..14,18..20} (16 alike) : DataTypeConversion  OutDataTypeStr=double  RndMeth=Nearest  SaturateOnIntegerOverflow=off
  Data Type Conversion{11,15..17,21..22} (6 alike) : DataTypeConversion  OutDataTypeStr=single  RndMeth=Nearest  SaturateOnIntegerOverflow=off
  Demux : Demux  Outputs=6
  Mux : Mux  Inputs=6
  Switch : Switch  Criteria=u2 ~= 0  SaturateOnIntegerOverflow=off  InputSameDT=off
  Switch1 : Switch  Criteria=u2 ~= 0  SaturateOnIntegerOverflow=off  InputSameDT=off
  mechanical_system : Subsystem
  pmsm : Subsystem
  torque_calculation : Subsystem
  outputs : Outport
  wires:
  reset_integrators/1 -> mechanical_system/1(reset), pmsm/1(reset)
  Data Type Conversion4/1 -> Switch1/3, Switch/3  "omega_mech"
  Switch/1 -> pmsm/13(omega_mech)
  reciprocal_J/1 -> Data Type Conversion14/1
  pmsm/2(psi_d) -> torque_calculation/2(psi_d)
  Data Type Conversion5/1 -> mechanical_system/6(load_torque)  "load_torque"
  Data Type Conversion7/1 -> pmsm/7(reciprocal_L_d)
  Switch1/1 -> Data Type Conversion17/1
  Data Type Conversion9/1 -> pmsm/6(psi_pm)
  R1/1 -> Data Type Conversion6/1
  Data Type Conversion6/1 -> pmsm/8(R1)
  pmsm/3(psi_q) -> torque_calculation/3(psi_q)
  Data Type Conversion10/1 -> pmsm/12(polepairs), torque_calculation/4(polepairs)
  Data Type Conversion2/1 -> pmsm/2(u_d)  "u_d"
  Data Type Conversion12/1 -> mechanical_system/3(mu)
  simulate_mechanical/1 -> Switch1/2, Switch/2
  M_n0/1 -> Data Type Conversion13/1
  Data Type Conversion14/1 -> mechanical_system/5(reciprocal_J)
  torque_calculation/1(M_Mi) -> mechanical_system/2(M_Mi), Data Type Conversion16/1
  mu/1 -> Data Type Conversion12/1
  psi_pm/1 -> Data Type Conversion9/1
  Data Type Conversion13/1 -> mechanical_system/4(M_n0)
  reciprocal_L_d/1 -> Data Type Conversion7/1
  Data Type Conversion8/1 -> pmsm/9(reciprocal_L_q)
  reciprocal_L_q/1 -> Data Type Conversion8/1
  polepairs/1 -> Data Type Conversion10/1
  Data Type Conversion3/1 -> pmsm/3(u_q)  "u_q"
  mechanical_system/1(omega_mech) -> Switch/1, Switch1/1
  pmsm/4(I_q) -> torque_calculation/5(I_q), Data Type Conversion15/1  "i_q"
  pmsm/1(I_d) -> torque_calculation/1(I_d), Data Type Conversion11/1  "i_d"
  Data Type Conversion17/1 -> Mux/6  "omega_mech"
  Data Type Conversion16/1 -> Mux/5  "M_Mi"
  Data Type Conversion15/1 -> Mux/2  "i_q"
  Data Type Conversion11/1 -> Mux/1  "i_d"
  Demux/1 -> Data Type Conversion2/1
  Demux/2 -> Data Type Conversion3/1
  Demux/5 -> Data Type Conversion4/1
  Demux/6 -> Data Type Conversion5/1
  inputs/1 -> Demux/1
  Mux/1 -> outputs/1
  Demux/3 -> Data Type Conversion1/1
  Demux/4 -> Data Type Conversion18/1
  Data Type Conversion1/1 -> pmsm/4(u_x)  "u_x"
  Data Type Conversion18/1 -> pmsm/5(u_y)  "u_y"
  reciprocal_L_x/1 -> Data Type Conversion19/1
  reciprocal_L_y/1 -> Data Type Conversion20/1
  Data Type Conversion19/1 -> pmsm/10(reciprocal_L_x)
  Data Type Conversion20/1 -> pmsm/11(reciprocal_L_y)
  Data Type Conversion21/1 -> Mux/3  "i_x"
  Data Type Conversion22/1 -> Mux/4  "i_y"
  pmsm/6(I_y) -> Data Type Conversion22/1
  pmsm/5(I_x) -> Data Type Conversion21/1

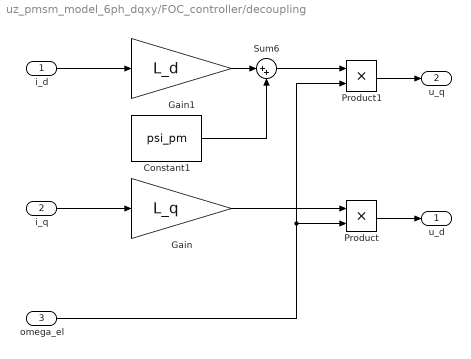
== system uz_pmsm_model_6ph_dqxy/FOC_controller/decoupling ==
  i_d : Inport
  i_q : Inport  Port=2
  omega_el : Inport  Port=3
  Constant1 : Constant  Value=psi_pm  SampleTime=-1
  Gain : Gain  Gain=L_q
  Gain1 : Gain  Gain=L_d
  Product : Product
  Product1 : Product
  Sum6 : Sum  Inputs=|++
  u_d : Outport
  u_q : Outport  Port=2
  wires:
  Gain/1 -> Product/1
  omega_el/1 -> Product1/2, Product/2
  Product1/1 -> u_q/1
  i_d/1 -> Gain1/1
  Product/1 -> u_d/1
  Gain1/1 -> Sum6/1
  i_q/1 -> Gain/1
  Constant1/1 -> Sum6/2
  Sum6/1 -> Product1/1

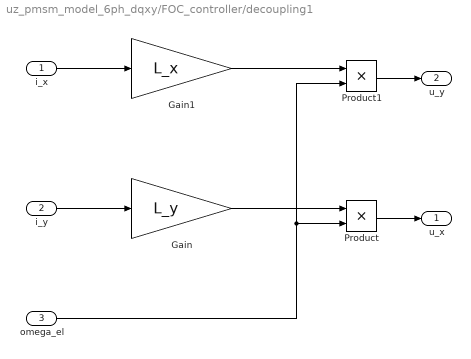
== system uz_pmsm_model_6ph_dqxy/FOC_controller/decoupling1 ==
  i_x : Inport
  i_y : Inport  Port=2
  omega_el : Inport  Port=3
  Gain : Gain  Gain=L_y
  Gain1 : Gain  Gain=L_x
  Product : Product
  Product1 : Product
  u_x : Outport
  u_y : Outport  Port=2
  wires:
  Gain/1 -> Product/1
  omega_el/1 -> Product1/2, Product/2
  Product1/1 -> u_y/1
  i_x/1 -> Gain1/1
  Product/1 -> u_x/1
  i_y/1 -> Gain/1
  Gain1/1 -> Product1/1

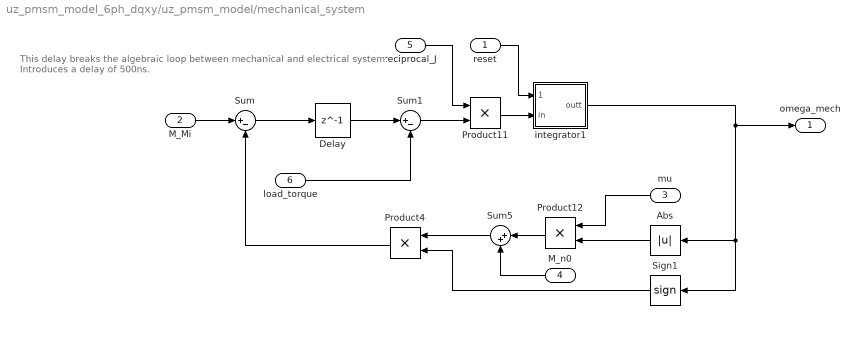
== system uz_pmsm_model_6ph_dqxy/uz_pmsm_model/mechanical_system ==
  note: This delay breaks the algebraic loop between mechanical and electrical system.
      | Introduces a delay of 500ns.
  reset : Inport
  M_Mi : Inport  Port=2
  mu : Inport  Port=3
  M_n0 : Inport  Port=4
  reciprocal_J : Inport  Port=5
  load_torque : Inport  Port=6
  Abs : Abs  SaturateOnIntegerOverflow=off
  Delay : Delay  DelayLength=1
  Product11 : Product
  Product12 : Product
  Product4 : Product
  Sign1 : Signum
  Sum : Sum  Inputs=|+-
  Sum1 : Sum  Inputs=|+-
  Sum5 : Sum  Inputs=|++
  integrator1 : Subsystem
  omega_mech : Outport
  wires:
  Product11/1 -> integrator1/2(in)
  Sum5/1 -> Product4/1
  Sign1/1 -> Product4/2
  integrator1/1(outt) -> Sign1/1, Abs/1, omega_mech/1
  Abs/1 -> Product12/2
  reset/1 -> integrator1/1(reset)
  Product12/1 -> Sum5/1
  mu/1 -> Product12/1
  M_n0/1 -> Sum5/2
  reciprocal_J/1 -> Product11/1
  M_Mi/1 -> Sum/1
  Sum1/1 -> Product11/2
  load_torque/1 -> Sum1/2
  Sum/1 -> Delay/1
  Product4/1 -> Sum/2
  Delay/1 -> Sum1/1

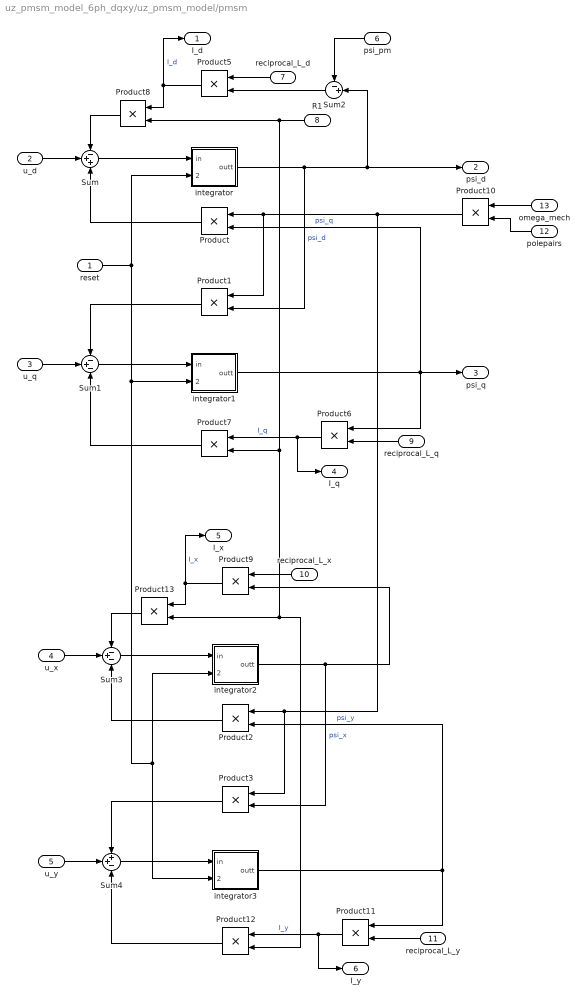
== system uz_pmsm_model_6ph_dqxy/uz_pmsm_model/pmsm ==
  reset : Inport
  u_d : Inport  Port=2
  u_q : Inport  Port=3
  u_x : Inport  Port=4
  u_y : Inport  Port=5
  psi_pm : Inport  Port=6
  reciprocal_L_d : Inport  Port=7
  R1 : Inport  Port=8
  reciprocal_L_q : Inport  Port=9
  reciprocal_L_x : Inport  Port=10
  reciprocal_L_y : Inport  Port=11
  polepairs : Inport  Port=12
  omega_mech : Inport  Port=13
  Product{,1..3,5..13} (13 alike) : Product
  Sum : Sum  Inputs=-++
  Sum1 : Sum  Inputs=-+-
  Sum2 : Sum  Inputs=-+|
  Sum3 : Sum  Inputs=-+-
  Sum4 : Sum  Inputs=++-
  integrator : Subsystem
  integrator1 : Subsystem
  integrator2 : Subsystem
  integrator3 : Subsystem
  I_d : Outport
  psi_d : Outport  Port=2
  psi_q : Outport  Port=3
  I_q : Outport  Port=4
  I_x : Outport  Port=5
  I_y : Outport  Port=6
  wires:
  omega_mech/1 -> Product10/1
  u_q/1 -> Sum1/2
  Product/1 -> Sum/3
  Product5/1 -> I_d/1, Product8/1  "I_d"
  reciprocal_L_d/1 -> Product5/1
  integrator1/1(outt) -> Product6/1, Product/2, psi_q/1  "psi_q"
  u_d/1 -> Sum/2
  Product1/1 -> Sum1/1
  Sum/1 -> integrator/1(in)
  psi_pm/1 -> Sum2/1
  Product6/1 -> I_q/1, Product7/1  "I_q"
  integrator/1(outt) -> psi_d/1, Sum2/2, Product1/2  "psi_d"
  Sum2/1 -> Product5/2
  Product8/1 -> Sum/1
  polepairs/1 -> Product10/2
  reciprocal_L_q/1 -> Product6/2
  Product7/1 -> Sum1/3
  Sum1/1 -> integrator1/1(in)
  reciprocal_L_x/1 -> Product9/1
  integrator2/1(outt) -> Product9/2, Product3/2  "psi_x"
  Product11/1 -> I_y/1, Product12/1  "I_y"
  Product3/1 -> Sum4/1
  Product10/1 -> Product3/1, Product2/1, Product1/1, Product/1
  reciprocal_L_y/1 -> Product11/2
  R1/1 -> Product13/2, Product12/2, Product7/2, Product8/2
  reset/1 -> integrator3/2(reset), integrator2/2(reset), integrator1/2(reset), integrator/2(reset)
  Product13/1 -> Sum3/1
  u_x/1 -> Sum3/2
  Sum4/1 -> integrator3/1(in)
  Product12/1 -> Sum4/3
  Product2/1 -> Sum3/3
  u_y/1 -> Sum4/2
  Product9/1 -> I_x/1, Product13/1  "I_x"
  Sum3/1 -> integrator2/1(in)
  integrator3/1(outt) -> Product11/1, Product2/2  "psi_y"

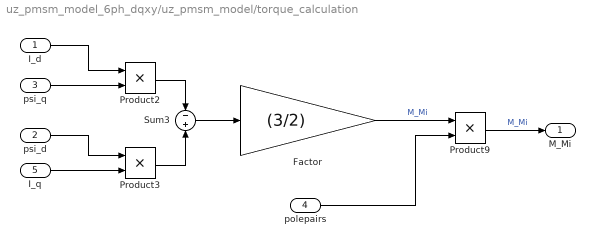
== system uz_pmsm_model_6ph_dqxy/uz_pmsm_model/torque_calculation ==
  I_d : Inport
  psi_d : Inport  Port=2
  psi_q : Inport  Port=3
  polepairs : Inport  Port=4
  I_q : Inport  Port=5
  Factor : Gain  Gain=(3/2)
  Product2 : Product
  Product3 : Product
  Product9 : Product
  Sum3 : Sum  Inputs=-|+
  M_Mi : Outport
  wires:
  Sum3/1 -> Factor/1
  Product3/1 -> Sum3/2
  Product2/1 -> Sum3/1
  psi_q/1 -> Product2/2
  psi_d/1 -> Product3/1
  I_d/1 -> Product2/1
  I_q/1 -> Product3/2
  Product9/1 -> M_Mi/1  "M_Mi"
  polepairs/1 -> Product9/2
  Factor/1 -> Product9/1  "M_Mi"

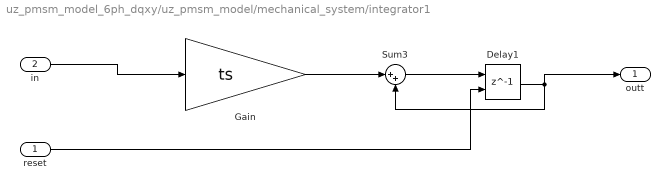
== system uz_pmsm_model_6ph_dqxy/uz_pmsm_model/mechanical_system/integrator1 ==
  reset : Inport
  in : Inport  Port=2
  Delay1 : Delay  DelayLength=1  ExternalReset=Level
      settings: InputPortMap=u0,r5
  Gain : Gain  Gain=ts  OutDataTypeStr=double
  Sum3 : Sum  Inputs=|++  OutDataTypeStr=double
  outt : Outport
  wires:
  in/1 -> Gain/1
  Gain/1 -> Sum3/1
  reset/1 -> Delay1/2
  Sum3/1 -> Delay1/1
  Delay1/1 -> Sum3/2, outt/1

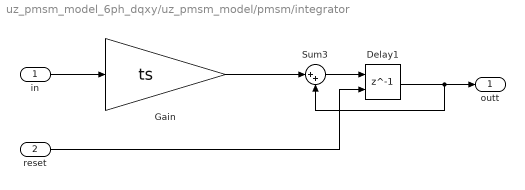
== system uz_pmsm_model_6ph_dqxy/uz_pmsm_model/pmsm/integrator ==
  in : Inport
  reset : Inport  Port=2
  Delay1 : Delay  DelayLength=1  ExternalReset=Level
      settings: InputPortMap=u0,r5
  Gain : Gain  Gain=ts  OutDataTypeStr=double
  Sum3 : Sum  Inputs=|++  OutDataTypeStr=double
  outt : Outport
  wires:
  reset/1 -> Delay1/2
  Gain/1 -> Sum3/1
  in/1 -> Gain/1
  Delay1/1 -> outt/1, Sum3/2
  Sum3/1 -> Delay1/1

== system uz_pmsm_model_6ph_dqxy/uz_pmsm_model/pmsm/integrator1 ==
  in : Inport
  reset : Inport  Port=2
  Delay1 : Delay  DelayLength=1  ExternalReset=Level
      settings: InputPortMap=u0,r5
  Gain : Gain  Gain=ts  OutDataTypeStr=double
  Sum3 : Sum  Inputs=|++  OutDataTypeStr=double
  outt : Outport
  wires:
  in/1 -> Gain/1
  Gain/1 -> Sum3/1
  reset/1 -> Delay1/2
  Delay1/1 -> Sum3/2, outt/1
  Sum3/1 -> Delay1/1

== system uz_pmsm_model_6ph_dqxy/uz_pmsm_model/pmsm/integrator2 ==
  in : Inport
  reset : Inport  Port=2
  Delay1 : Delay  DelayLength=1  ExternalReset=Level
      settings: InputPortMap=u0,r5
  Gain : Gain  Gain=ts  OutDataTypeStr=double
  Sum3 : Sum  Inputs=|++  OutDataTypeStr=double
  outt : Outport
  wires:
  reset/1 -> Delay1/2
  Gain/1 -> Sum3/1
  in/1 -> Gain/1
  Delay1/1 -> outt/1, Sum3/2
  Sum3/1 -> Delay1/1

== system uz_pmsm_model_6ph_dqxy/uz_pmsm_model/pmsm/integrator3 ==
  in : Inport
  reset : Inport  Port=2
  Delay1 : Delay  DelayLength=1  ExternalReset=Level
      settings: InputPortMap=u0,r5
  Gain : Gain  Gain=ts  OutDataTypeStr=double
  Sum3 : Sum  Inputs=|++  OutDataTypeStr=double
  outt : Outport
  wires:
  in/1 -> Gain/1
  Gain/1 -> Sum3/1
  reset/1 -> Delay1/2
  Delay1/1 -> Sum3/2, outt/1
  Sum3/1 -> Delay1/1
